simulink model "Phase1_Mark2"  (R2024b)
settings: Solver=ode23tb  StartTime=0.0  StopTime=inf  FixedStep=.001  RelTol=1e-1
model workspace (MAT data in the model file):
  A_mu = 10
  B_reff = 8.386
  CONVERTER_DATA = [0 0.1 0.2 0.3 0.4 0.5 0.6 0.7 0.8 0.81 0.82 0.83 ... (63 elements, 21x3)]
  Cps = 2
  Cz = 7766.25
  DOWN_TABLE = [0 0 0 0 0 0 5 5 7.5 7.5 15 15 ... (30 elements, 6x5)]
  DOWN_TH_BP = [0 5 40 50 90 100]
  D_reff = 0.25826
  EMAP = [-40 215 245 264 264 267 267 267 267 267 -44 117 ... (110 elements, 10x11)]
  F0z = [6086.4 4324.8]
  F_reff = 0.07394
  F_zmax = 10000
  F_zmin = 100
  F_zo = 4000
  Kz = 48000
  MF : object (value not decoded)
  NCyl = 6
  NE_VEC = [800 1200 1600 2000 2400 2800 3200 3600 4000 4400 4800]
  Pstd = 101325
  Rair = 287
  SUS : object (value not decoded)
  TH_VEC = [0; 20; 30; 40; 50; 60; 70; 80; 90; 100]
  TWAITdn = 1.25
  TWAITup = 0.1
  Tin = [1 2 3 4 5 6 7 8 9 10 2 2 ... (20 elements, 10x2)]
  Tstd = 293.15
  UP_TABLE = [7.5 7.5 15 25 40 40 25 25 35 45 70 80 ... (30 elements, 6x5)]
  UP_TH_BP = [0 25 35 50 90 100]
  VEH : object (value not decoded)
  V_o = 16.7
  V_xlow = 1
  Vd = 0.00346
  WH : object (value not decoded)
  a = 1.515
  alpha_max = 1.5
  alpha_min = -1.5
  b = 1.504
  c_zo = 209651
  epsilon = 0.1
  f_air = [0 0 0 0 0 0 0 0 0 0 0 0 ... (256 elements, 16x16)]
  f_co = [0 0 0 0 0 0 0 0 0 0 0 0 ... (256 elements, 16x16)]
  f_co2 = [0 0 0 0 0 0 0 0 0 0 0 0 ... (256 elements, 16x16)]
  f_eff = [352.135682859 352.135682859 320.724378192 303.655312657 295.930136708 291.240087194 291.240271258 291.240312459 291.240275452 291.240198499 291.240100781 291.240018769 ... (256 elements, 16x16)]
  f_fuel = [0 0 0 0 0 0 0 0 0 0 0 0 ... (256 elements, 16x16)]
  f_hc = [0 0 0 0 0 0 0 0 0 0 0 0 ... (256 elements, 16x16)]
  f_nox = [0 0 0 0 0 0 0 0 0 0 0 0 ... (256 elements, 16x16)]
  f_pm = [0 0 0 0 0 0 0 0 0 0 0 0 ... (256 elements, 16x16)]
  f_susp_axl_bp = [1 2]
  f_susp_dz_bp = [-4 -0.14 -0.13 -0.12 -0.11 -0.1 -0.09 -0.08 -0.07 -0.06 -0.05 -0.04 ... (31 elements, 1x31)]
  f_susp_dzdot_bp = [-4 -0.14 -0.13 -0.12 -0.11 -0.1 -0.09 -0.08 -0.07 -0.06 -0.05 -0.04 ... (31 elements, 1x31)]
  f_susp_fmz = [-213379.591456 -28099.591456 -27619.591456 -27139.591456 -26659.591456 -26179.591456 -25699.591456 -25219.591456 -24739.591456 -24259.591456 -23779.591456 -23299.591456 ... (468968 elements, 31x31x61x2x4)]
  f_susp_geom = [-0.832564012244 0.043269987756 0.045538987756 0.047807987756 0.050076987756 0.052345987756 0.054614987756 0.056883987756 0.059152987756 0.061421987756 0.063690987756 0.065959987756 ... (11346 elements, 31x61x2x3)]
  f_susp_strgdelta_bp = [-0.523598775598 -0.506145483078 -0.488692190558 -0.471238898038 -0.453785605519 -0.436332312999 -0.418879020479 -0.401425727959 -0.383972435439 -0.366519142919 -0.349065850399 -0.331612557879 ... (61 elements, 1x61)]
  f_tbrake = [0 76.8593923996 105.140482948 131.533638111 157.926793274 176.658631717 176.65727296 176.656856686 176.656879077 176.657093756 176.657404516 176.65772406 ... (256 elements, 16x16)]
  f_tbrake_n_bpt = [0 649.519052838 912.419621844 1175.32019085 1438.22075986 1701.12132886 1964.02189787 2226.92246687 2489.82303588 2752.72360489 3015.62417389 3278.5247429 ... (16 elements, 1x16)]
  f_tbrake_t_bpt = [0 34.6410161514 61.0341713143 87.4273264773 113.82048164 140.213636803 166.606791966 192.999947129 219.393102292 245.786257455 272.179412618 298.572567781 ... (16 elements, 1x16)]
  f_texh = [766.752464599 766.752464599 786.17542386 801.679939032 884.591982581 910.574397722 910.571871054 910.570774534 910.570601632 910.570821151 910.571247242 910.571639815 ... (256 elements, 16x16)]
  f_twc_eff_co = [0.17 0.25 0.45 0.99 0.99 0.99 0.99]
  f_twc_eff_hc = [0.21 0.375 0.75 0.98 0.98 0.98 0.98]
  f_twc_eff_lam = [0.909090909 0.944055944 0.979020979 1 1.013986014 1.048951049 1.083916084]
  f_twc_eff_nox = [0.98 0.98 0.98 0.97 0.05 0.02 0]
  h = 0.134
  k_z = 50
  kappa_max = 1.5
  kappa_min = -1.5
  lam_Cx = 1
  lam_Cy = 1
  lam_Cz = 1
  lam_Ex = 1
  lam_Ey = 1
  lam_F_zo = 1
  lam_Hx = 1
  lam_Hy = 1
  lam_Kxkappa = 1
  lam_Kyalpha = 1
  lam_Kygamma = 1
  lam_Kzgamma = 1
  lam_Mr = 1
  lam_Mx = 1
  lam_My = 1
  lam_S = 1
  lam_VMx = 1
  lam_Vx = 1
  lam_Vy = 1
  lam_Vykappa = 1
  lam_muV = 0
  lam_mux = 1
  lam_muy = 1
  lam_t = 1
  lam_xalpha = 1
  lam_ykappa = 1
  numWheel = 4
  p_Cx1 = 1.579
  p_Cy1 = 1.3332
  p_Dx1 = 1.0422
  p_Dx2 = -0.08285
  p_Dx3 = 0
  p_Dy1 = 0.8784
  p_Dy2 = -0.06445
  p_Dy3 = 0
  p_Ex1 = 0.11185
  p_Ex2 = 0.3127
  p_Ex3 = 0
  p_Ex4 = 0.001603
  p_Ey1 = -0.8227
  p_Ey2 = -0.6062
  p_Ey3 = 0.09825
  p_Ey4 = -6.546
  p_Ey5 = 0
  p_Fz1 = 0.7098
  p_Hx1 = 0.00021585
  p_Hx2 = 0.0011538
  p_Hy1 = -0.0018043
  p_Hy2 = 0.003518
  p_Kx1 = 21.69
  p_Kx2 = 13.774
  p_Kx3 = -0.4119
  p_Ky1 = -15.314
  p_Ky2 = 1.7044
  p_Ky3 = 0.36986
  p_Ky4 = 1.9896
  p_Ky5 = 0
  p_Ky6 = -0.9004
  p_Ky7 = -0.2328
  p_Vx1 = 1.5973e-05
  p_Vx2 = 0.0001043
  p_Vy1 = -0.006642
  p_Vy2 = 0.03597
  p_Vy3 = -0.1621
  p_Vy4 = -0.4908
  p_pmx1 = 0
  p_px1 = -0.3489
  p_px2 = 0.382
  p_px3 = -0.09634
  p_px4 = 0.06447
  p_py1 = -0.6249
  p_py2 = -0.06535
  p_py3 = -0.1668
  p_py4 = 0.2834
  p_py5 = 0
  path : object (value not decoded)
  pio = 220000
  q_Fcx = 0
  q_Fz2 = 15.4
  q_Fzy = 0
  q_reo = 0.9974
  q_sx1 = -0.007764
  q_sx10 = 0.2824
  q_sx11 = 5.349
  q_sx12 = 0
  q_sx13 = 0
  q_sx14 = 0
  q_sx2 = 1.1915
  q_sx3 = 0.013948
  q_sx4 = 4.912
  q_sx5 = 1.02
  q_sx6 = 22.83
  q_sx7 = 0.7104
  q_sx8 = -0.023393
  q_sx9 = 0.6581
  q_sy1 = 0.00702
  q_sy2 = 0
  q_sy3 = 0.001515
  q_sy4 = 8.514e-05
  q_sy5 = 0
  q_sy6 = 0
  q_sy7 = 0.9008
  q_sy8 = -0.4089
  q_v1 = 0.0007742
  q_v2 = 0.04667
  r_Bx1 = 12.531
  r_Bx2 = 9.532
  r_Bx3 = 0
  r_By1 = 10.615
  r_By2 = 7.705
  r_By3 = 3.433e-06
  r_By4 = 0
  r_Cx1 = 1.019
  r_Cy1 = 1.0585
  r_Ex1 = -0.4487
  r_Ex2 = -0.4726
  r_Ey1 = 0.3132
  r_Ey2 = 7.63e-06
  r_Hx1 = 0.0002374
  r_Hy1 = 0.011646
  r_Hy2 = 7.63e-06
  r_Vy1 = 0.05654
  r_Vy2 = 7.63e-06
  r_Vy3 = 0
  r_Vy4 = 99.9
  r_Vy5 = 2
  r_Vy6 = 15.814
  r_o = 0.3135
  reqTmaxT = [nan 0.285774810084 0.647179872268 nan nan nan nan nan nan nan nan nan ... (168 elements, 21x8)]
  vehSpd = [0 2.77777777778 5.55555555556 8.33333333333 11.1111111111 13.8888888889 16.6666666667 19.4444444444 22.2222222222 25 27.7777777778 30.5555555556 ... (21 elements, 1x21)]
  vehWidth = 2
  w = 1
symbols that are objects in the model workspace (value not decoded): VEH
undefined symbols (not defined in the file or in its folder): Fzz, Fzzdot, InertFrm, pFz, psi, vdyntiremask, x_o, zdotFz, zFz
(part 24 of 24)

== system Phase1_Mark2/Vehicle Body 3DOF External Longitudinal Wheels/Dual/Vehicle Body 3DOF Dual Track/Signal Routing/Signal Routing Dual/Lateral 3DOF/Hard Point Coordinate Transform Rear Right/Hard Point Coordinate Transform External Displacement/wxR/Subsystem ==
  A : Inport
  B : Inport  Port=2
  Demux : Demux  Outputs=3
  Demux1 : Demux  Outputs=3
  Mux : Mux  Inputs=3
  i x j : Product  InputSameDT=on  SaturateOnIntegerOverflow=on  OutDataTypeStr=Inherit: Same as first input
  j x k : Product  InputSameDT=on  SaturateOnIntegerOverflow=on  OutDataTypeStr=Inherit: Same as first input
  k x i : Product  InputSameDT=on  SaturateOnIntegerOverflow=on  OutDataTypeStr=Inherit: Same as first input
  Out1 : Outport  VectorParamsAs1DForOutWhenUnconnected=off
  wires:
  Demux1/3 -> j x k/2
  Demux/2 -> j x k/1
  Demux/3 -> k x i/1
  Demux1/1 -> k x i/2
  Demux1/2 -> i x j/2
  Demux/1 -> i x j/1
  i x j/1 -> Mux/3
  k x i/1 -> Mux/2
  j x k/1 -> Mux/1
  B/1 -> Demux1/1
  A/1 -> Demux/1
  Mux/1 -> Out1/1

== system Phase1_Mark2/Vehicle Body 3DOF External Longitudinal Wheels/Dual/Vehicle Body 3DOF Dual Track/Signal Routing/Signal Routing Dual/Lateral 3DOF/Hard Point Coordinate Transform Rear Right/Hard Point Coordinate Transform External Displacement/wxR/Subsystem1 ==
  A : Inport
  B : Inport  Port=2
  Demux : Demux  Outputs=3
  Demux1 : Demux  Outputs=3
  Mux : Mux  Inputs=3
  i x k : Product  InputSameDT=on  SaturateOnIntegerOverflow=on  OutDataTypeStr=Inherit: Same as first input
  j x i : Product  InputSameDT=on  SaturateOnIntegerOverflow=on  OutDataTypeStr=Inherit: Same as first input
  k x j : Product  InputSameDT=on  SaturateOnIntegerOverflow=on  OutDataTypeStr=Inherit: Same as first input
  Out1 : Outport  VectorParamsAs1DForOutWhenUnconnected=off
  wires:
  j x i/1 -> Mux/3
  i x k/1 -> Mux/2
  k x j/1 -> Mux/1
  Mux/1 -> Out1/1
  Demux1/1 -> j x i/2
  Demux/2 -> j x i/1
  Demux1/3 -> i x k/2
  Demux/1 -> i x k/1
  Demux1/2 -> k x j/2
  Demux/3 -> k x j/1
  B/1 -> Demux1/1
  A/1 -> Demux/1

== system Phase1_Mark2/Vehicle Body 3DOF External Longitudinal Wheels/Dual/Vehicle Body 3DOF Dual Track/Signal Routing/Signal Routing Dual/Lateral 3DOF/Hitch Coordinate Transform/Hard Point Coordinate Transform External Displacement/Rotation Angles to Direction Cosine Matrix/Create 3x3 Matrix ==
  M11 : Inport  PortDimensions=1
  M12 : Inport  Port=2  PortDimensions=1
  M13 : Inport  Port=3  PortDimensions=1
  M21 : Inport  Port=4  PortDimensions=1
  M22 : Inport  Port=5  PortDimensions=1
  M23 : Inport  Port=6  PortDimensions=1
  M31 : Inport  Port=7  PortDimensions=1
  M32 : Inport  Port=8  PortDimensions=1
  M33 : Inport  Port=9  PortDimensions=1
  Reshape (9) to [3x3] column-major : Reshape  OutputDimensionality=Customize  OutputDimensions=[3,3]
  Vector Concatenate : Concatenate  NumInputs=9
  Matrix : Outport  PortDimensions=[3 3]  VectorParamsAs1DForOutWhenUnconnected=off
  wires:
  M33/1 -> Vector Concatenate/9
  M23/1 -> Vector Concatenate/8
  M13/1 -> Vector Concatenate/7
  M32/1 -> Vector Concatenate/6
  Reshape (9) to [3x3] column-major/1 -> Matrix/1
  M22/1 -> Vector Concatenate/5
  M12/1 -> Vector Concatenate/4
  M31/1 -> Vector Concatenate/3
  M21/1 -> Vector Concatenate/2
  M11/1 -> Vector Concatenate/1
  Vector Concatenate/1 -> Reshape (9) to [3x3] column-major/1

== system Phase1_Mark2/Vehicle Body 3DOF External Longitudinal Wheels/Dual/Vehicle Body 3DOF Dual Track/Signal Routing/Signal Routing Dual/Lateral 3DOF/Hitch Coordinate Transform/Hard Point Coordinate Transform External Displacement/wxR/Subsystem ==
  A : Inport
  B : Inport  Port=2
  Demux : Demux  Outputs=3
  Demux1 : Demux  Outputs=3
  Mux : Mux  Inputs=3
  i x j : Product  InputSameDT=on  SaturateOnIntegerOverflow=on  OutDataTypeStr=Inherit: Same as first input
  j x k : Product  InputSameDT=on  SaturateOnIntegerOverflow=on  OutDataTypeStr=Inherit: Same as first input
  k x i : Product  InputSameDT=on  SaturateOnIntegerOverflow=on  OutDataTypeStr=Inherit: Same as first input
  Out1 : Outport  VectorParamsAs1DForOutWhenUnconnected=off
  wires:
  Demux1/3 -> j x k/2
  Demux/2 -> j x k/1
  Demux/3 -> k x i/1
  Demux1/1 -> k x i/2
  Demux1/2 -> i x j/2
  Demux/1 -> i x j/1
  i x j/1 -> Mux/3
  k x i/1 -> Mux/2
  j x k/1 -> Mux/1
  B/1 -> Demux1/1
  A/1 -> Demux/1
  Mux/1 -> Out1/1

== system Phase1_Mark2/Vehicle Body 3DOF External Longitudinal Wheels/Dual/Vehicle Body 3DOF Dual Track/Signal Routing/Signal Routing Dual/Lateral 3DOF/Hitch Coordinate Transform/Hard Point Coordinate Transform External Displacement/wxR/Subsystem1 ==
  A : Inport
  B : Inport  Port=2
  Demux : Demux  Outputs=3
  Demux1 : Demux  Outputs=3
  Mux : Mux  Inputs=3
  i x k : Product  InputSameDT=on  SaturateOnIntegerOverflow=on  OutDataTypeStr=Inherit: Same as first input
  j x i : Product  InputSameDT=on  SaturateOnIntegerOverflow=on  OutDataTypeStr=Inherit: Same as first input
  k x j : Product  InputSameDT=on  SaturateOnIntegerOverflow=on  OutDataTypeStr=Inherit: Same as first input
  Out1 : Outport  VectorParamsAs1DForOutWhenUnconnected=off
  wires:
  j x i/1 -> Mux/3
  i x k/1 -> Mux/2
  k x j/1 -> Mux/1
  Mux/1 -> Out1/1
  Demux1/1 -> j x i/2
  Demux/2 -> j x i/1
  Demux1/3 -> i x k/2
  Demux/1 -> i x k/1
  Demux1/2 -> k x j/2
  Demux/3 -> k x j/1
  B/1 -> Demux1/1
  A/1 -> Demux/1

== system Phase1_Mark2/Longitudinal Wheels 4DOF/Tires/Fiala/Fiala Tire/Wheel Module/Clutch/Clutch Partitioned Parameters/Clutch/detectLockup/Friction Mode Logic/Lockup Detection/Friction Calc ==
  Tout : Inport
  Unary Minus : UnaryMinus
  Friction Torque : Outport  InitialOutput=0  VectorParamsAs1DForOutWhenUnconnected=off
  wires:
  Tout/1 -> Unary Minus/1
  Unary Minus/1 -> Friction Torque/1

== system Phase1_Mark2/Longitudinal Wheels 4DOF/Tires/Fiala/Fiala Tire/Wheel Module/Clutch/Clutch Partitioned Parameters/Clutch/detectLockup/Friction Mode Logic/Lockup Detection/Required Friction for Lockup ==
  Friction Torque : Inport
  Max Friction Torque : Inport  Port=2
  Abs : Abs  ZeroCross=off
  Relational Operator : RelationalOperator  Operator=<=  OutDataTypeStr=boolean  ZeroCross=off
  okay : Outport  InitialOutput=0  VectorParamsAs1DForOutWhenUnconnected=off
  wires:
  Max Friction Torque/1 -> Relational Operator/2
  Abs/1 -> Relational Operator/1
  Relational Operator/1 -> okay/1
  Friction Torque/1 -> Abs/1

== system Phase1_Mark2/Longitudinal Wheels 4DOF/Tires/Fiala/Fiala Tire/Wheel Module/Clutch/Clutch Scalar Parameters/Clutch/detectLockup/Friction Mode Logic/Lockup Detection/Friction Calc ==
  Tout : Inport
  Unary Minus : UnaryMinus
  Friction Torque : Outport  InitialOutput=0  VectorParamsAs1DForOutWhenUnconnected=off
  wires:
  Tout/1 -> Unary Minus/1
  Unary Minus/1 -> Friction Torque/1

== system Phase1_Mark2/Longitudinal Wheels 4DOF/Tires/Fiala/Fiala Tire/Wheel Module/Clutch/Clutch Scalar Parameters/Clutch/detectLockup/Friction Mode Logic/Lockup Detection/Required Friction for Lockup ==
  Friction Torque : Inport
  Max Friction Torque : Inport  Port=2
  Abs : Abs  ZeroCross=off
  Relational Operator : RelationalOperator  Operator=<=  OutDataTypeStr=boolean  ZeroCross=off
  okay : Outport  InitialOutput=0  VectorParamsAs1DForOutWhenUnconnected=off
  wires:
  Max Friction Torque/1 -> Relational Operator/2
  Abs/1 -> Relational Operator/1
  Relational Operator/1 -> okay/1
  Friction Torque/1 -> Abs/1

== system Phase1_Mark2/Longitudinal Wheels 4DOF/Tires/MF/Combined Slip Wheel 2DOF/Wheel Module/Clutch/Clutch Partitioned Parameters/Clutch/detectLockup/Friction Mode Logic/Lockup Detection/Friction Calc ==
  Tout : Inport
  Unary Minus : UnaryMinus
  Friction Torque : Outport  InitialOutput=0  VectorParamsAs1DForOutWhenUnconnected=off
  wires:
  Tout/1 -> Unary Minus/1
  Unary Minus/1 -> Friction Torque/1

== system Phase1_Mark2/Longitudinal Wheels 4DOF/Tires/MF/Combined Slip Wheel 2DOF/Wheel Module/Clutch/Clutch Partitioned Parameters/Clutch/detectLockup/Friction Mode Logic/Lockup Detection/Required Friction for Lockup ==
  Friction Torque : Inport
  Max Friction Torque : Inport  Port=2
  Abs : Abs  ZeroCross=off
  Relational Operator : RelationalOperator  Operator=<=  OutDataTypeStr=boolean  ZeroCross=off
  okay : Outport  InitialOutput=0  VectorParamsAs1DForOutWhenUnconnected=off
  wires:
  Max Friction Torque/1 -> Relational Operator/2
  Abs/1 -> Relational Operator/1
  Relational Operator/1 -> okay/1
  Friction Torque/1 -> Abs/1

== system Phase1_Mark2/Longitudinal Wheels 4DOF/Tires/MF/Combined Slip Wheel 2DOF/Wheel Module/Clutch/Clutch Scalar Parameters/Clutch/detectLockup/Friction Mode Logic/Lockup Detection/Friction Calc ==
  Tout : Inport
  Unary Minus : UnaryMinus
  Friction Torque : Outport  InitialOutput=0  VectorParamsAs1DForOutWhenUnconnected=off
  wires:
  Tout/1 -> Unary Minus/1
  Unary Minus/1 -> Friction Torque/1

== system Phase1_Mark2/Longitudinal Wheels 4DOF/Tires/MF/Combined Slip Wheel 2DOF/Wheel Module/Clutch/Clutch Scalar Parameters/Clutch/detectLockup/Friction Mode Logic/Lockup Detection/Required Friction for Lockup ==
  Friction Torque : Inport
  Max Friction Torque : Inport  Port=2
  Abs : Abs  ZeroCross=off
  Relational Operator : RelationalOperator  Operator=<=  OutDataTypeStr=boolean  ZeroCross=off
  okay : Outport  InitialOutput=0  VectorParamsAs1DForOutWhenUnconnected=off
  wires:
  Max Friction Torque/1 -> Relational Operator/2
  Abs/1 -> Relational Operator/1
  Relational Operator/1 -> okay/1
  Friction Torque/1 -> Abs/1

== system Phase1_Mark2/Vehicle Body 3DOF External Longitudinal Wheels/Bicycle/Vehicle Body 3DOF Single Track/Signal Routing/Signal Routing/Lateral 3DOF/Hard Point Coordinate Transform Geometric/Hard Point Coordinate Transform External Displacement Beta/Body Slip/div0protect - abs poly/Compare To Constant ==
  u : Inport
  Compare : RelationalOperator  OutDataTypeStr=boolean  ZeroCross=off
  Constant : Constant  DisableCoverage=on  Value=const  OutDataTypeStr=Inherit: Inherit via back propagation
  y : Outport
  wires:
  u/1 -> Compare/1
  Constant/1 -> Compare/2
  Compare/1 -> y/1

== system Phase1_Mark2/Vehicle Body 3DOF External Longitudinal Wheels/Bicycle/Vehicle Body 3DOF Single Track/Signal Routing/Signal Routing/Lateral 3DOF/Hard Point Coordinate Transform Geometric/Hard Point Coordinate Transform External Displacement Beta/Body Slip/div0protect - abs poly/Compare To Constant1 ==
  u : Inport
  Compare : RelationalOperator  Operator=<=  OutDataTypeStr=boolean  ZeroCross=off
  Constant : Constant  DisableCoverage=on  Value=const  OutDataTypeStr=Inherit: Inherit via back propagation
  y : Outport
  wires:
  u/1 -> Compare/1
  Constant/1 -> Compare/2
  Compare/1 -> y/1

== system Phase1_Mark2/Vehicle Body 3DOF External Longitudinal Wheels/Bicycle/Vehicle Body 3DOF Single Track/Signal Routing/Signal Routing Dual/Lateral 3DOF/Hard Point Coordinate Transform Geometric/Hard Point Coordinate Transform External Displacement Beta/Body Slip/div0protect - abs poly/Compare To Constant ==
  u : Inport
  Compare : RelationalOperator  OutDataTypeStr=boolean  ZeroCross=off
  Constant : Constant  DisableCoverage=on  Value=const  OutDataTypeStr=Inherit: Inherit via back propagation
  y : Outport
  wires:
  u/1 -> Compare/1
  Constant/1 -> Compare/2
  Compare/1 -> y/1

== system Phase1_Mark2/Vehicle Body 3DOF External Longitudinal Wheels/Bicycle/Vehicle Body 3DOF Single Track/Signal Routing/Signal Routing Dual/Lateral 3DOF/Hard Point Coordinate Transform Geometric/Hard Point Coordinate Transform External Displacement Beta/Body Slip/div0protect - abs poly/Compare To Constant1 ==
  u : Inport
  Compare : RelationalOperator  Operator=<=  OutDataTypeStr=boolean  ZeroCross=off
  Constant : Constant  DisableCoverage=on  Value=const  OutDataTypeStr=Inherit: Inherit via back propagation
  y : Outport
  wires:
  u/1 -> Compare/1
  Constant/1 -> Compare/2
  Compare/1 -> y/1

== system Phase1_Mark2/Vehicle Body 3DOF External Longitudinal Wheels/Dual/Vehicle Body 3DOF Dual Track/Signal Routing/Signal Routing/Lateral 3DOF/Hard Point Coordinate Transform Geometric/Hard Point Coordinate Transform External Displacement Beta/Body Slip/div0protect - abs poly/Compare To Constant ==
  u : Inport
  Compare : RelationalOperator  OutDataTypeStr=boolean  ZeroCross=off
  Constant : Constant  DisableCoverage=on  Value=const  OutDataTypeStr=Inherit: Inherit via back propagation
  y : Outport
  wires:
  u/1 -> Compare/1
  Constant/1 -> Compare/2
  Compare/1 -> y/1

== system Phase1_Mark2/Vehicle Body 3DOF External Longitudinal Wheels/Dual/Vehicle Body 3DOF Dual Track/Signal Routing/Signal Routing/Lateral 3DOF/Hard Point Coordinate Transform Geometric/Hard Point Coordinate Transform External Displacement Beta/Body Slip/div0protect - abs poly/Compare To Constant1 ==
  u : Inport
  Compare : RelationalOperator  Operator=<=  OutDataTypeStr=boolean  ZeroCross=off
  Constant : Constant  DisableCoverage=on  Value=const  OutDataTypeStr=Inherit: Inherit via back propagation
  y : Outport
  wires:
  u/1 -> Compare/1
  Constant/1 -> Compare/2
  Compare/1 -> y/1

== system Phase1_Mark2/Vehicle Body 3DOF External Longitudinal Wheels/Dual/Vehicle Body 3DOF Dual Track/Signal Routing/Signal Routing Dual/Lateral 3DOF/Hard Point Coordinate Transform Geometric/Hard Point Coordinate Transform External Displacement Beta/Body Slip/div0protect - abs poly/Compare To Constant ==
  u : Inport
  Compare : RelationalOperator  OutDataTypeStr=boolean  ZeroCross=off
  Constant : Constant  DisableCoverage=on  Value=const  OutDataTypeStr=Inherit: Inherit via back propagation
  y : Outport
  wires:
  u/1 -> Compare/1
  Constant/1 -> Compare/2
  Compare/1 -> y/1

== system Phase1_Mark2/Vehicle Body 3DOF External Longitudinal Wheels/Dual/Vehicle Body 3DOF Dual Track/Signal Routing/Signal Routing Dual/Lateral 3DOF/Hard Point Coordinate Transform Geometric/Hard Point Coordinate Transform External Displacement Beta/Body Slip/div0protect - abs poly/Compare To Constant1 ==
  u : Inport
  Compare : RelationalOperator  Operator=<=  OutDataTypeStr=boolean  ZeroCross=off
  Constant : Constant  DisableCoverage=on  Value=const  OutDataTypeStr=Inherit: Inherit via back propagation
  y : Outport
  wires:
  u/1 -> Compare/1
  Constant/1 -> Compare/2
  Compare/1 -> y/1

== matlab function Phase1_Mark2/Longitudinal Wheels 4DOF/Tires/Fiala/Fiala Tire/Fiala/Rolling/Mapped/MATLAB Function ==
  data: omega input; My output; Fz input; Vx input; VxMy parameter; FzMy parameter; MyMap parameter; FZMAX parameter
function My = MappedMy(omega,Fz,Vx,VxMy, FzMy, MyMap, FZMAX)%#codegen
coder.allowpcode('plain')
My = automltirelongMyMapped(omega,Fz,Vx,VxMy,FzMy,MyMap,FZMAX);
end

== stateflow chart Phase1_Mark2/Longitudinal Wheels 4DOF/Tires/MF/Combined Slip Wheel 2DOF/Wheel Module/Clutch/Clutch Partitioned Parameters/Clutch ==
  settings: updateMethod=CONTINUOUS
  state yn = detectSlip(Tout,Tfmaxs) [function]
  state Slipping
  state yn = detectLockup(Tout,Tfmaxs) [function]
  state Locked
  (default) -> Slipping : {Slipping.omegaWheel = omegao;}
  Slipping -> Locked : [detectLockup(Tout, Tfmaxs) && (abs(Omega)<=OmegaTol)]
  Locked -> Slipping : [detectSlip(Tout,Tfmaxs)]
      | {
      | Slipping.omegaWheel = 0;
      | }
  data: yn function_output; Tout function_input double size=1; Tfmaxs function_input double size=1; sf_internal_action_state_placeholder_data local double size=1 =0; omegaWheel local; yn function_output; Tout function_input double size=1; Tfmaxs function_input double size=1; sf_internal_action_state_placeholder_data local double size=1 =0; Tout input double; Tfmaxs input double; Tfmaxk input double; Omega output double; Omegadot output double; Myb output double; ReactionTorque output double; omegao parameter double; OmegaTol parameter; BrkTrq output double

== stateflow chart Phase1_Mark2/Longitudinal Wheels 4DOF/Tires/MF/Combined Slip Wheel 2DOF/Wheel Module/Clutch/Clutch Scalar Parameters/Clutch ==
  settings: updateMethod=CONTINUOUS
  state yn = detectSlip(Tout,Tfmaxs) [function]
  state Slipping
  state yn = detectLockup(Tout,Tfmaxs) [function]
  state Locked
  (default) -> Slipping : {Slipping.omegaWheel = omegao;}
  Slipping -> Locked : [detectLockup(Tout, Tfmaxs) && (abs(Omega)<=OmegaTol)]
  Locked -> Slipping : [detectSlip(Tout,Tfmaxs)]
      | {
      | Slipping.omegaWheel = 0;
      | }
  data: yn function_output; Tout function_input double size=1; Tfmaxs function_input double size=1; sf_internal_action_state_placeholder_data local double size=1 =0; omegaWheel local; yn function_output; Tout function_input double size=1; Tfmaxs function_input double size=1; sf_internal_action_state_placeholder_data local double size=1 =0; Tout input double; Tfmaxs input double; Tfmaxk input double; Omega output double; Omegadot output double; Myb output double; ReactionTorque output double; omegao parameter double; OmegaTol parameter; BrkTrq output double

== matlab function Phase1_Mark2/Vehicle Body 3DOF External Longitudinal Wheels/Bicycle/Vehicle Body 3DOF Single Track/Signal Routing/Signal Routing/state2bus/COMB2I ==
  data: x input size=4; y output size=2
function y = fcn(x)%#codegen
coder.allowpcode('plain')
y = automlvehb2i(x);

== matlab function Phase1_Mark2/Vehicle Body 3DOF External Longitudinal Wheels/Bicycle/Vehicle Body 3DOF Single Track/Signal Routing/Signal Routing Dual/state2bus/COMB2I ==
  data: x input size=4; y output size=2
function y = fcn(x)%#codegen
coder.allowpcode('plain')
y = automlvehb2i(x);

== matlab function Phase1_Mark2/Vehicle Body 3DOF External Longitudinal Wheels/Bicycle/Vehicle Body 3DOF Single Track/vehicle model ==
  data: delta_f input; delta_r input; mu input; a parameter; b parameter; h parameter; d parameter; w parameter; m parameter; NF parameter; NR parameter; Izz parameter; g parameter; Fxtire_sat parameter size=1; Fytire_sat parameter size=1; trackMode parameter; inputMode parameter; xdot_tol parameter; Fznom parameter size=1; F_f input; F_r input; F_ext input size=3; M_ext input size=3; Fh input size=3; Mh input size=3; Cy_f input; Cy_r input; dh input; hl input; hh input; yOut output size=3; FBody output size=3; MBody output size=3; FOut output; FTire output; Fg output size=3; wheelInfo output; stateDer output size=4; stateVec input size=4; status output size=1
function [yOut,FBody,MBody,FOut,FTire,Fg,wheelInfo,stateDer,status] = fcn(delta_f,delta_r,mu,a,b,h,d,w,m,NF,NR,Izz,g,Fxtire_sat,Fytire_sat,trackMode,inputMode,xdot_tol,Fznom,F_f,F_r,F_ext,M_ext,Fh,Mh,Cy_f,Cy_r,dh,hl,hh,stateVec)%#codegen
coder.allowpcode('plain')
switch trackMode
    case 1
       [yOut,FBody,MBody,FOut,FTire,Fg,wheelInfo,stateDer,status] = automlvehdynbicycle(delta_f,delta_r,mu,a,b,h,m,NF,NR,Izz,g,Fxtire_sat,Fytire_sat,inputMode,xdot_tol,Fznom,F_f,F_r,F_ext,M_ext,Fh,Mh,Cy_f,Cy_r,dh,hh,stateVec);
    case 2
       [yOut,FBody,MBody,FOut,FTire,Fg,wheelInfo,stateDer,status] = automlvehdyndualtrack(delta_f,delta_r,mu,a,b,h,d,w,m,NF,NR,Izz,g,Fxtire_sat,Fytire_sat,inputMode,xdot_tol,Fznom,F_f,F_r,F_ext,M_ext,Fh,Mh,Cy_f,Cy_r,dh,hl,hh,stateVec);
end
end

== matlab function Phase1_Mark2/Vehicle Body 3DOF External Longitudinal Wheels/Dual/Vehicle Body 3DOF Dual Track/Signal Routing/Signal Routing/state2bus/COMB2I ==
  data: x input size=4; y output size=2
function y = fcn(x)%#codegen
coder.allowpcode('plain')
y = automlvehb2i(x);

== matlab function Phase1_Mark2/Vehicle Body 3DOF External Longitudinal Wheels/Dual/Vehicle Body 3DOF Dual Track/Signal Routing/Signal Routing Dual/state2bus/COMB2I ==
  data: x input size=4; y output size=2
function y = fcn(x)%#codegen
coder.allowpcode('plain')
y = automlvehb2i(x);

== matlab function Phase1_Mark2/Vehicle Body 3DOF External Longitudinal Wheels/Dual/Vehicle Body 3DOF Dual Track/vehicle model ==
  data: delta_f input; delta_r input; mu input; a parameter; b parameter; h parameter; d parameter; w parameter; m parameter; NF parameter; NR parameter; Izz parameter; g parameter; Fxtire_sat parameter size=1; Fytire_sat parameter size=1; trackMode parameter; inputMode parameter; xdot_tol parameter; Fznom parameter size=1; F_f input; F_r input; F_ext input size=3; M_ext input size=3; Fh input size=3; Mh input size=3; Cy_f input; Cy_r input; dh input; hl input; hh input; yOut output size=3; FBody output size=3; MBody output size=3; FOut output; FTire output; Fg output size=3; wheelInfo output; stateDer output size=4; stateVec input size=4; status output size=1
function [yOut,FBody,MBody,FOut,FTire,Fg,wheelInfo,stateDer,status] = fcn(delta_f,delta_r,mu,a,b,h,d,w,m,NF,NR,Izz,g,Fxtire_sat,Fytire_sat,trackMode,inputMode,xdot_tol,Fznom,F_f,F_r,F_ext,M_ext,Fh,Mh,Cy_f,Cy_r,dh,hl,hh,stateVec)%#codegen
coder.allowpcode('plain')
switch trackMode
    case 1
       [yOut,FBody,MBody,FOut,FTire,Fg,wheelInfo,stateDer,status] = automlvehdynbicycle(delta_f,delta_r,mu,a,b,h,m,NF,NR,Izz,g,Fxtire_sat,Fytire_sat,inputMode,xdot_tol,Fznom,F_f,F_r,F_ext,M_ext,Fh,Mh,Cy_f,Cy_r,dh,hh,stateVec);
    case 2
       [yOut,FBody,MBody,FOut,FTire,Fg,wheelInfo,stateDer,status] = automlvehdyndualtrack(delta_f,delta_r,mu,a,b,h,d,w,m,NF,NR,Izz,g,Fxtire_sat,Fytire_sat,inputMode,xdot_tol,Fznom,F_f,F_r,F_ext,M_ext,Fh,Mh,Cy_f,Cy_r,dh,hl,hh,stateVec);
end
end

== matlab function Phase1_Mark2/Longitudinal Wheels 4DOF/Tires/Fiala/Fiala Tire/Fiala/MATLAB Function ==
  data: Vx input; Fx output; Vy input; gamma input; psidot input; prs input; Fz input; rhoz input; ScaleFctr input; kappa input; alpha input; Fy output; Mx output; Mz output; Re output; UNLOADED_RADIUS parameter; WIDTH parameter; CAMMIN parameter; CAMMAX parameter; PRESMIN parameter; PRESMAX parameter; FZMIN parameter; FZMAX parameter; KPUMIN parameter; KPUMAX parameter; ALPMIN parameter; ALPMAX parameter; Ckappa parameter; Calpha parameter; Cgamma parameter; muMax parameter; muMin parameter; aMy parameter; bMy parameter; alphaMy parameter; cMy parameter; betaMy parameter; bMz parameter
function [Fx,Fy,Mx,Mz,Re] = fialaTire(Vx,Vy,gamma,psidot,prs,Fz,rhoz,ScaleFctr,...
                                          kappa, alpha,...
                                          UNLOADED_RADIUS, WIDTH,...
                                          CAMMIN, CAMMAX, PRESMIN, PRESMAX, FZMIN, FZMAX,...
                                           KPUMIN, KPUMAX, ALPMIN, ALPMAX,...
                                          Ckappa, Calpha, Cgamma,muMax,muMin,...
                                          aMy, bMy, alphaMy, cMy, betaMy, bMz)

%#codegen
coder.allowpcode('plain');
[Fx,Fy,Mx,~,Mz,Re,~,~] = vdynfialatire(Vx,Vy,gamma,0,psidot,prs,Fz,rhoz,ScaleFctr,...
                                         kappa,alpha,0,...
                                         UNLOADED_RADIUS,WIDTH,...
                                         0,...
                                         CAMMIN,CAMMAX,PRESMIN,PRESMAX,FZMIN,FZMAX,...
                                         KPUMIN,KPUMAX, ALPMIN, ALPMAX,...
                                         Ckappa,Calpha,Cgamma,muMax,muMin,...
                                         aMy,bMy,cMy,alphaMy,betaMy,bMz);
end

== matlab function Phase1_Mark2/Vehicle Signal Routing/For 3D Visualization ==
  data: angles output size=3; angleIn input size=3; GeomXYZ output size=3; GemoXYZIn input size=3; Ground input size=4; trackW parameter; wheelB parameter
function [angles,GeomXYZ]= three26(angleIn, GemoXYZIn, Ground,trackW, wheelB)%#codegen
coder.allowpcode('plain')
% Copyright 2018 The MathWorks, Inc.
[angles,GeomXYZ]= vdynthree2six(angleIn, GemoXYZIn, Ground,trackW, wheelB);

== stateflow chart Phase1_Mark2/Longitudinal Wheels 4DOF/Tires/Fiala/Fiala Tire/Wheel Module/Clutch/Clutch Partitioned Parameters/Clutch ==
  settings: updateMethod=CONTINUOUS
  state yn = detectSlip(Tout,Tfmaxs) [function]
  state Slipping
  state yn = detectLockup(Tout,Tfmaxs) [function]
  state Locked
  (default) -> Slipping : {Slipping.omegaWheel = omegao;}
  Slipping -> Locked : [detectLockup(Tout, Tfmaxs) && (abs(Omega)<=OmegaTol)]
  Locked -> Slipping : [detectSlip(Tout,Tfmaxs)]
      | {
      | Slipping.omegaWheel = 0;
      | }
  data: yn function_output; Tout function_input double size=1; Tfmaxs function_input double size=1; sf_internal_action_state_placeholder_data local double size=1 =0; omegaWheel local; yn function_output; Tout function_input double size=1; Tfmaxs function_input double size=1; sf_internal_action_state_placeholder_data local double size=1 =0; Tout input double; Tfmaxs input double; Tfmaxk input double; Omega output double; Omegadot output double; Myb output double; ReactionTorque output double; omegao parameter double; OmegaTol parameter; BrkTrq output double

== matlab function Phase1_Mark2/Longitudinal Wheels 4DOF/Tires/Fiala/Fiala Tire/Wheel Module/Brakes/Drum Brake/Drum Brake/Drum Brake Torque Calculation ==
  data: P input; Ba input; T output; mu input; a input; c input; r input; theta1 input; theta2 input
function T=CalcDrumShoeTorque(P,Ba,mu,a,c,r,theta1,theta2)

   %Convert angles from deg to rad
   theta1=theta1.*pi./180.;
   theta2=theta2.*pi./180.;
     
   %Calculate torque terms 
   sigma=cos(theta2)-cos(theta1);
   
   Numerator=pi.*mu.*c.*r.*sigma.*Ba.^2;
   
   Denominator1=2.*mu.*(-2.*r.*sigma-a.*(cos(theta1).^2-cos(theta2).^2));

   Denominator2=a.*(2.*theta1-2.*theta2-sin(2.*theta1)+sin(2.*theta2));
    
   %Right shoe torque
   Tr=P.*Numerator./(Denominator1+Denominator2);
    
   %Left shoe torque
   Tl=P.*Numerator./(-Denominator1+Denominator2);

   T=Tr+Tl;
   
end

== stateflow chart Phase1_Mark2/Longitudinal Wheels 4DOF/Tires/Fiala/Fiala Tire/Wheel Module/Clutch/Clutch Scalar Parameters/Clutch ==
  settings: updateMethod=CONTINUOUS
  state yn = detectSlip(Tout,Tfmaxs) [function]
  state Slipping
  state yn = detectLockup(Tout,Tfmaxs) [function]
  state Locked
  (default) -> Slipping : {Slipping.omegaWheel = omegao;}
  Slipping -> Locked : [detectLockup(Tout, Tfmaxs) && (abs(Omega)<=OmegaTol)]
  Locked -> Slipping : [detectSlip(Tout,Tfmaxs)]
      | {
      | Slipping.omegaWheel = 0;
      | }
  data: yn function_output; Tout function_input double size=1; Tfmaxs function_input double size=1; sf_internal_action_state_placeholder_data local double size=1 =0; omegaWheel local; yn function_output; Tout function_input double size=1; Tfmaxs function_input double size=1; sf_internal_action_state_placeholder_data local double size=1 =0; Tout input double; Tfmaxs input double; Tfmaxk input double; Omega output double; Omegadot output double; Myb output double; ReactionTorque output double; omegao parameter double; OmegaTol parameter; BrkTrq output double

== matlab function Phase1_Mark2/Longitudinal Wheels 4DOF/Tires/MF/Combined Slip Wheel 2DOF/Magic Tire Const Input/Magic Tire Const Input ==
  data: Omega input; Vx input; Vy input; psidot input; Gamma input; TirePrs input; ScaleFactors input; rhoz input; plySteer parameter; turnslip parameter; Fx output; Fy output; FzTire output; Mx output; My output; Mz output; Re output; Kappa output; Alpha output; sig_x output; sig_y output; PRESMAX parameter; PRESMIN parameter; FZMAX parameter; FZMIN parameter; VXLOW parameter; KPUMAX parameter; KPUMIN parameter; ALPMAX parameter; ALPMIN parameter; CAMMIN parameter; CAMMAX parameter; LONGVL parameter; UNLOADED_RADIUS parameter; RIM_RADIUS parameter; NOMPRES parameter; FNOMIN parameter; VERTICAL_STIFFNESS parameter; DREFF parameter; BREFF parameter; FREFF parameter; Q_RE0 parameter; Q_V1 parameter; Q_V2 parameter; Q_FZ1 parameter; Q_FZ2 parameter; Q_FCX parameter; Q_FCY parameter; PFZ1 parameter; Q_FCY2 parameter; BOTTOM_OFFST parameter; BOTTOM_STIFF parameter; PCX1 parameter; PDX1 parameter; PDX2 parameter; PDX3 parameter; PEX1 parameter; PEX2 parameter; PEX3 parameter; PEX4 parameter; PKX1 parameter; PKX2 parameter; PKX3 parameter; PHX1 parameter; PHX2 parameter; PVX1 parameter; PVX2 parameter; PPX1 parameter; PPX2 parameter; PPX3 parameter; PPX4 parameter; RBX1 parameter; RBX2 parameter; RBX3 parameter; RCX1 parameter; REX1 parameter; REX2 parameter; RHX1 parameter; QSX1 parameter; QSX2 parameter; QSX3 parameter; QSX4 parameter; QSX5 parameter; QSX6 parameter; QSX7 parameter; QSX8 parameter; QSX9 parameter; QSX10 parameter; QSX11 parameter; PPMX1 parameter; PCY1 parameter; PDY1 parameter; PDY2 parameter; PDY3 parameter; PEY1 parameter; PEY2 parameter; PEY3 parameter; PEY4 parameter; PEY5 parameter; PKY1 parameter; PKY2 parameter; PKY3 parameter; PKY4 parameter; PKY5 parameter; PKY6 parameter; PKY7 parameter; PHY1 parameter; PHY2 parameter; PVY1 parameter; PVY2 parameter; PVY3 parameter; PVY4 parameter; PPY1 parameter; PPY2 parameter; PPY3 parameter; PPY4 parameter; PPY5 parameter; RBY1 parameter; RBY2 parameter; RBY3 parameter; RBY4 parameter; RCY1 parameter; REY1 parameter; REY2 parameter; RHY1 parameter; RHY2 parameter; RVY1 parameter; RVY2 parameter; RVY3 parameter; RVY4 parameter; RVY5 parameter; RVY6 parameter; QSY1 parameter; QSY2 parameter; QSY3 parameter; QSY4 parameter; QSY5 parameter; QSY6 parameter; QSY7 parameter; QSY8 parameter; QBZ1 parameter; QBZ2 parameter; QBZ3 parameter; QBZ4 parameter; QBZ5 parameter; QBZ6 parameter; QBZ9 parameter; QBZ10 parameter; QCZ1 parameter; QDZ1 parameter; QDZ2 parameter; QDZ3 parameter; QDZ4 parameter; QDZ6 parameter; QDZ7 parameter; QDZ8 parameter; QDZ9 parameter; QDZ10 parameter; QDZ11 parameter; QEZ1 parameter; QEZ2 parameter; QEZ3 parameter; QEZ4 parameter; QEZ5 parameter; QHZ1 parameter; QHZ2 parameter; QHZ3 parameter; QHZ4 parameter; PPZ1 parameter; PPZ2 parameter; SSZ1 parameter; SSZ2 parameter; SSZ3 parameter; SSZ4 parameter; PDXP1 parameter; PDXP2 parameter; PDXP3 parameter; PKYP1 parameter; PDYP1 parameter; PDYP2 parameter; PDYP3 parameter; PDYP4 parameter; PHYP1 parameter; PHYP2 parameter; PHYP3 parameter; PHYP4 parameter; PECP1 parameter; PECP2 parameter; QDTP1 parameter; QCRP1 parameter; QCRP2 parameter; QBRP1 parameter; QDRP1 parameter; QDRP2 parameter; WIDTH parameter; Q_RA1 parameter; Q_RA2 parameter; Q_RB1 parameter; Q_RB2 parameter; QSX12 parameter; QSX13 parameter; QSX14 parameter; a output; b output; Q_FZ3 parameter; LONGITUDINAL_STIFFNESS parameter; LATERAL_STIFFNESS parameter; PCFX1 parameter; PCFX2 parameter; PCFX3 parameter; PCFY1 parameter; PCFY2 parameter; PCFY3 parameter; Fx_ext input; Fy_ext input; Fz_ext input; vdynMF parameter size=279; vertType input; Q_CAM1 parameter; Q_CAM2 parameter; Q_CAM3 parameter; Q_FYS1 parameter; Q_FYS2 parameter; Q_FYS3 parameter; ASPECT_RATIO parameter; RL output; RadialDeflct output; Tw output
% Copyright 2018-2023 The MathWorks, Inc.
function [Fx,Fy,FzTire,Mx,My,Mz,Re,Kappa,Alpha,sig_x,sig_y,a,b,RL,RadialDeflct,Tw] = magictire(Omega,Vx,Vy,psidot, Gamma,TirePrs,ScaleFactors,rhoz,plySteer,turnslip, ...
    PRESMAX,...
    PRESMIN,...
    FZMAX,...
    FZMIN,...
    VXLOW,...
    KPUMAX,...
    KPUMIN,...
    ALPMAX,...
    ALPMIN,...
    CAMMIN,...
    CAMMAX,...
    LONGVL,...
    UNLOADED_RADIUS,...    
    RIM_RADIUS,...
    NOMPRES,...
    FNOMIN,...
    VERTICAL_STIFFNESS,...% vertical
    DREFF,...
    BREFF,...
    FREFF,...
    Q_RE0,...
    Q_V1,...
    Q_V2,...
    Q_FZ1,...
    Q_FZ2,...
    Q_FCX,...
    Q_FCY,...
    PFZ1,...
    Q_FCY2,...
    BOTTOM_OFFST,...
    BOTTOM_STIFF,...
    PCX1,...% longitudinal
    PDX1,...
    PDX2,...
    PDX3,...
    PEX1,...
    PEX2,...
    PEX3,...
    PEX4,...
    PKX1,...
    PKX2,...
    PKX3,...
    PHX1,...
    PHX2,...
    PVX1,...
    PVX2,...
    PPX1,...
    PPX2,...
    PPX3,...
    PPX4,...
    RBX1,...
    RBX2,...
    RBX3,...
    RCX1,...
    REX1,...
    REX2,...
    RHX1,...
    QSX1,...% overturning
    QSX2,...
    QSX3,...
    QSX4,...
    QSX5,...
    QSX6,...
    QSX7,...
    QSX8,...
    QSX9,...
    QSX10,...
    QSX11,...
    PPMX1,...
    PCY1,...% lateral
    PDY1,...
    PDY2,...
    PDY3,...
    PEY1,...
    PEY2,...
    PEY3,...
    PEY4,...
    PEY5,...
    PKY1,...
    PKY2,...
    PKY3,...
    PKY4,...
    PKY5,...
    PKY6,...
    PKY7,...
    PHY1,...
    PHY2,...
    PVY1,...
    PVY2,...
    PVY3,...
    PVY4,...
    PPY1,...
    PPY2,...
    PPY3,...
    PPY4,...
    PPY5,...
    RBY1,...
    RBY2,...
    RBY3,...
    RBY4,...
    RCY1,...
    REY1,...
    REY2,...
    RHY1,...
    RHY2,...
    RVY1,...
    RVY2,...
    RVY3,...
    RVY4,...
    RVY5,...
    RVY6,...
    QSY1,...% rolling
    QSY2,...
    QSY3,...
    QSY4,...
    QSY5,...
    QSY6,...
    QSY7,...
    QSY8,...
    QBZ1,...
    QBZ2,...
    QBZ3,...
    QBZ4,...
    QBZ5,...
    QBZ6,...
    QBZ9,...
    QBZ10,...
    QCZ1,...
    QDZ1,...
    QDZ2,...
    QDZ3,...
    QDZ4,...
    QDZ6,...
    QDZ7,...
    QDZ8,...
    QDZ9,...
    QDZ10,...
    QDZ11,...
    QEZ1,...
    QEZ2,...
    QEZ3,...
    QEZ4,...
    QEZ5,...
    QHZ1,...
    QHZ2,...
    QHZ3,...
    QHZ4,...
    PPZ1,...
    PPZ2,...
    SSZ1,...
    SSZ2,...
    SSZ3,...
    SSZ4,...
    PDXP1,...% turn slip
    PDXP2,...
    PDXP3,...
    PKYP1,...
    PDYP1,...
    PDYP2,...
    PDYP3,...
    PDYP4,...
    PHYP1,...
    PHYP2,...
    PHYP3,...
    PHYP4,...
    PECP1,...
    PECP2,...
    QDTP1,...
    QCRP1,...% aligning moment
    QCRP2,...
    QBRP1,...
    QDRP1,...
    QDRP2,...
    WIDTH,...
    Q_RA1,... % contact patch
    Q_RA2,...
    Q_RB1,...
    Q_RB2,...
    QSX12,...
    QSX13,...
    QSX14,...
    Q_FZ3,...
    LONGITUDINAL_STIFFNESS,...% structural
    LATERAL_STIFFNESS,...
    PCFX1,...
    PCFX2,...
    PCFX3,...
    PCFY1,...
    PCFY2,...
    PCFY3,...
    Fx_ext,...
    Fy_ext,...
    Fz_ext,...
    vdynMF,...
    vertType, ...
    Q_CAM1, ...
    Q_CAM2, ...
    Q_CAM3, ...
    Q_FYS1, ...
    Q_FYS2, ...
    Q_FYS3, ...
    ASPECT_RATIO)
%#codegen
[Fx,Fy,FzTire,Mx,My,Mz,Re,Kappa,Alpha,sig_x,sig_y,a,b,RL,RadialDeflct,Tw] = vdyncsmtire(Omega,Vx,Vy,psidot,Gamma,TirePrs,ScaleFactors,rhoz,plySteer,turnslip,...
    PRESMAX,...
    PRESMIN,...
    FZMAX,...
    FZMIN,...
    VXLOW,...
    KPUMAX,...
    KPUMIN,...
    ALPMAX,...
    ALPMIN,...
    CAMMIN,...
    CAMMAX,...
    LONGVL,...
    UNLOADED_RADIUS,...
    RIM_RADIUS,...
    NOMPRES,...
    FNOMIN,...
    VERTICAL_STIFFNESS,...% vertical
    DREFF,...
    BREFF,...
    FREFF,...
    Q_RE0,...
    Q_V1,...
    Q_V2,...
    Q_FZ1,...
    Q_FZ2,...
    Q_FCX,...
    Q_FCY,...
    PFZ1,...
    Q_FCY2,...
    BOTTOM_OFFST,...
    BOTTOM_STIFF,...
    PCX1,...% longitudinal
    PDX1,...
    PDX2,...
    PDX3,...
    PEX1,...
    PEX2,...
    PEX3,...
    PEX4,...
    PKX1,...
    PKX2,...
    PKX3,...
    PHX1,...
    PHX2,...
    PVX1,...
    PVX2,...
    PPX1,...
    PPX2,...
    PPX3,...
    PPX4,...
    RBX1,...
    RBX2,...
    RBX3,...
    RCX1,...
    REX1,...
    REX2,...
    RHX1,...
    QSX1,...% overturning
    QSX2,...
    QSX3,...
    QSX4,...
    QSX5,...
    QSX6,...
    QSX7,...
    QSX8,...
    QSX9,...
    QSX10,...
    QSX11,...
    PPMX1,...
    PCY1,...% lateral
    PDY1,...
    PDY2,...
    PDY3,...
    PEY1,...
    PEY2,...
    PEY3,...
    PEY4,...
    PEY5,...
    PKY1,...
    PKY2,...
    PKY3,...
    PKY4,...
    PKY5,...
    PKY6,...
    PKY7,...
    PHY1,...
    PHY2,...
    PVY1,...
    PVY2,...
    PVY3,...
    PVY4,...
    PPY1,...
    PPY2,...
    PPY3,...
    PPY4,...
    PPY5,...
    RBY1,...
    RBY2,...
    RBY3,...
    RBY4,...
    RCY1,...
    REY1,...
    REY2,...
    RHY1,...
    RHY2,...
    RVY1,...
    RVY2,...
    RVY3,...
    RVY4,...
    RVY5,...
    RVY6,...
    QSY1,...% rolling
    QSY2,...
    QSY3,...
    QSY4,...
    QSY5,...
    QSY6,...
    QSY7,...
    QSY8,...
    QBZ1,...
    QBZ2,...
    QBZ3,...
    QBZ4,...
    QBZ5,...
    QBZ6,...
    QBZ9,...
    QBZ10,...
    QCZ1,...
    QDZ1,...
    QDZ2,...
    QDZ3,...
    QDZ4,...
    QDZ6,...
    QDZ7,...
    QDZ8,...
    QDZ9,...
    QDZ10,...
    QDZ11,...
    QEZ1,...
    QEZ2,...
    QEZ3,...
    QEZ4,...
    QEZ5,...
    QHZ1,...
    QHZ2,...
    QHZ3,...
    QHZ4,...
    PPZ1,...
    PPZ2,...
    SSZ1,...
    SSZ2,...
    SSZ3,...
    SSZ4,...
    PDXP1,...% turn slip
    PDXP2,...
    PDXP3,...
    PKYP1,...
    PDYP1,...
    PDYP2,...
    PDYP3,...
    PDYP4,...
    PHYP1,...
    PHYP2,...
    PHYP3,...
    PHYP4,...
    PECP1,...
    PECP2,...
    QDTP1,...
    QCRP1,...% aligning moment
    QCRP2,...
    QBRP1,...
    QDRP1,...
    QDRP2,...
    WIDTH,...
    Q_RA1,... % contact patch
    Q_RA2,...
    Q_RB1,...
    Q_RB2,...
    QSX12,...
    QSX13,...
    QSX14,...
    Q_FZ3,...
    LONGITUDINAL_STIFFNESS,...% structural
    LATERAL_STIFFNESS,...
    PCFX1,...
    PCFX2,...
    PCFX3,...
    PCFY1,...
    PCFY2,...
    PCFY3,...
    Fx_ext,...
    Fy_ext,...
    Fz_ext,...
    0,...
    0,...
    vdynMF,...
    vertType,...
    2,...
    Q_CAM1, ...
    Q_CAM2, ...
    Q_CAM3,...
    Q_FYS1, ...
    Q_FYS2, ...
    Q_FYS3, ...
    ASPECT_RATIO);
end

== matlab function Phase1_Mark2/Longitudinal Wheels 4DOF/Tires/MF/Combined Slip Wheel 2DOF/Wheel Module/Brakes/Drum Brake/Drum Brake/Drum Brake Torque Calculation ==
  data: P input; Ba input; T output; mu input; a input; c input; r input; theta1 input; theta2 input
function T=CalcDrumShoeTorque(P,Ba,mu,a,c,r,theta1,theta2)

   %Convert angles from deg to rad
   theta1=theta1.*pi./180.;
   theta2=theta2.*pi./180.;
     
   %Calculate torque terms 
   sigma=cos(theta2)-cos(theta1);
   
   Numerator=pi.*mu.*c.*r.*sigma.*Ba.^2;
   
   Denominator1=2.*mu.*(-2.*r.*sigma-a.*(cos(theta1).^2-cos(theta2).^2));

   Denominator2=a.*(2.*theta1-2.*theta2-sin(2.*theta1)+sin(2.*theta2));
    
   %Right shoe torque
   Tr=P.*Numerator./(Denominator1+Denominator2);
    
   %Left shoe torque
   Tl=P.*Numerator./(-Denominator1+Denominator2);

   T=Tr+Tl;
   
end

== matlab function Phase1_Mark2/Longitudinal Wheels 4DOF/Tires/Fiala/Fiala Tire/Fiala/Rolling/ISO/MATLAB Function ==
  data: Fz input; My output; omega input; Tamb input; Re input; Fpl parameter; Cr parameter; Kt parameter; Tmeas parameter; FZMIN parameter; FZMAX parameter; TMIN parameter; TMAX parameter
function My = ISOMy(Fz,omega,Tamb,Re,Fpl, Cr, Kt, Tmeas, FZMIN, FZMAX, TMIN, TMAX)%#codegen
coder.allowpcode('plain')
My = automltirelongMyISO(Fz,omega,Tamb,Fpl,Cr,Kt,Tmeas,Re,FZMIN,FZMAX,TMIN,TMAX);

== matlab function Phase1_Mark2/Longitudinal Wheels 4DOF/Tires/Fiala/Fiala Tire/Fiala/Rolling/MagicFormula/MATLAB Function ==
  data: Omega input; Fx input; My output; Fz input; Vx input; press input; gamma input; PRESMAX parameter size=1; FNOMIN parameter size=1; NOMPRES parameter size=1; QSY1 parameter size=1; QSY2 parameter size=1; QSY3 parameter size=1; QSY4 parameter size=1; QSY5 parameter size=1; QSY6 parameter size=1; QSY7 parameter size=1; QSY8 parameter size=1; lam_My parameter size=1; UNLOADED_RADIUS parameter size=1; FZMAX parameter size=1; PRESMIN parameter size=1
function My = MFMy(Omega,Fx,Fz,Vx,press,gamma,PRESMAX, FNOMIN, NOMPRES, QSY1, QSY2,...%#codegen
QSY3, QSY4, QSY5, QSY6, QSY7, QSY8, lam_My, UNLOADED_RADIUS, FZMAX, PRESMIN)
My = -automltirelongMy(Fx,Fz,Omega,Vx,press,FNOMIN, NOMPRES, QSY1, QSY2,...
    QSY3, QSY4,QSY5,QSY6,QSY7,QSY8,gamma,lam_My, UNLOADED_RADIUS,FZMAX,PRESMIN,PRESMAX);
end
